simulink model "regulator_P_simulink"  (R2025b)
settings: Solver=VariableStepAuto  StartTime=0.0  StopTime=150  RelTol=1e-3
values from neighbouring files (symbols this model uses):
  Kp_Bode = mnoznik*ZapasWzmocnieniaBezwymiarowy_bode    (= 3.22827114517)    [Regulator_P.m]
  Kp_Tau_T = (0.3)/(Kr*(tau/T))    [Regulator_P.m]
  L1 = [3]    [Regulator_P.m]
  M1 = conv(m4,m5)    [Regulator_P.m]
settings Model: LastModifiedBy=mefir

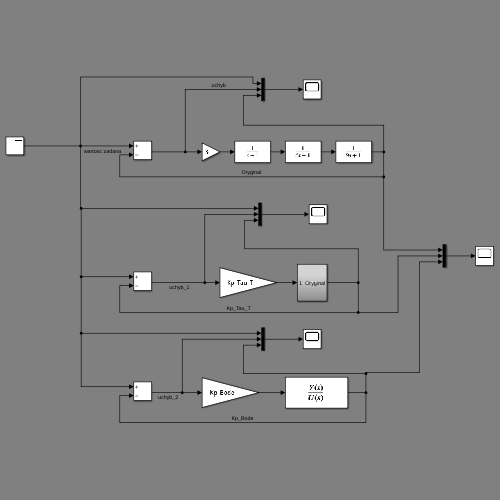
[thumbnail: Simulink's stored preview of the top-level diagram]
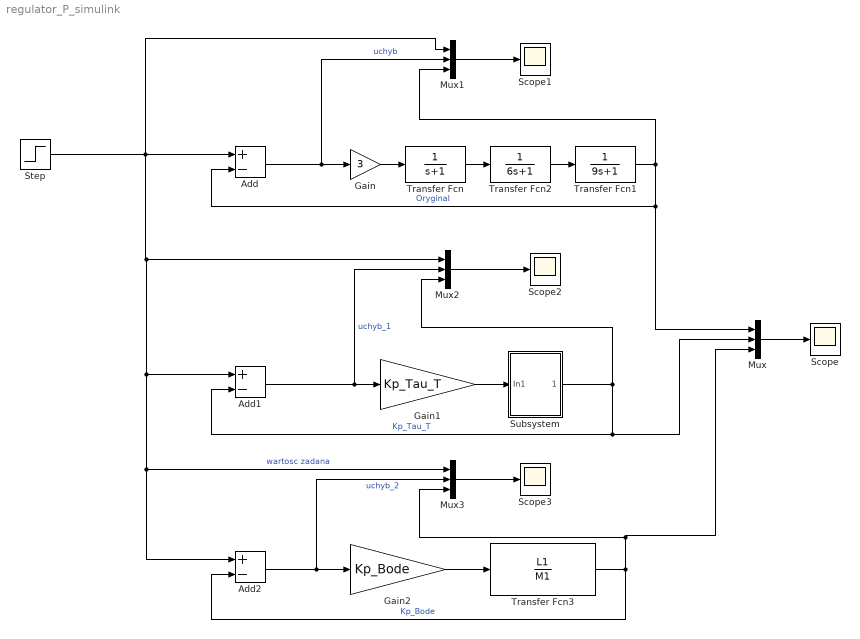
== system regulator_P_simulink ==
  Add : Sum  Inputs=+-
  Add1 : Sum  Inputs=+-
  Add2 : Sum  Inputs=+-
  Gain : Gain  Gain=3
  Gain1 : Gain  Gain=Kp_Tau_T
  Gain2 : Gain  Gain=Kp_Bode
  Mux{,1..3} (4 alike) : Mux  Inputs=3
  Scope{,1..3} (4 alike) : Scope
      Scope settings: ActiveDisplayYMinimum=-0.18004571836253325  ActiveDisplayYMaximum=1.6204114652627999
      Scope1 settings: ActiveDisplayYMinimum=-0.18004571836253325  ActiveDisplayYMaximum=1.6204114652627999
      Scope2 settings: ActiveDisplayYMinimum=-0.18004571836253325  ActiveDisplayYMaximum=1.6204114652627999  DataLoggingVariableName=ScopeData2
      Scope3 settings: ActiveDisplayYMinimum=-0.92077361092448817  ActiveDisplayYMaximum=2.8222475639378457  DataLoggingVariableName=ScopeData3
  Step : Step  Time=0  SampleTime=0
  Subsystem : Subsystem
  Transfer Fcn : TransferFcn  Denominator=[1 1]
  Transfer Fcn1 : TransferFcn  Denominator=[9 1]
  Transfer Fcn2 : TransferFcn  Denominator=[6 1]
  Transfer Fcn3 : TransferFcn  Numerator=L1  Denominator=M1
  wires:
  Transfer Fcn/1 -> Transfer Fcn2/1
  Transfer Fcn2/1 -> Transfer Fcn1/1
  Gain/1 -> Transfer Fcn/1
  Add/1 -> Mux1/2, Gain/1  "uchyb"
  Transfer Fcn1/1 -> Mux1/3, Mux/1, Add/2  "Oryginal"
  Add1/1 -> Mux2/2, Gain1/1  "uchyb_1"
  Gain1/1 -> Subsystem/1(In1)
  Subsystem/1(Oryginal) -> Mux2/3, Add1/2, Mux/2  "Kp_Tau_T"
  Step/1 -> Add/1, Mux2/1, Add1/1, Mux3/1, Add2/1, Mux1/1  "wartosc zadana"
  Add2/1 -> Mux3/2, Gain2/1  "uchyb_2"
  Transfer Fcn3/1 -> Add2/2, Mux3/3, Mux/3  "Kp_Bode"
  Mux/1 -> Scope/1
  Mux1/1 -> Scope1/1
  Gain2/1 -> Transfer Fcn3/1
  Mux2/1 -> Scope2/1
  Mux3/1 -> Scope3/1

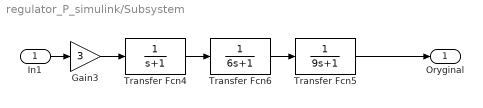
== system regulator_P_simulink/Subsystem ==
  In1 : Inport
  Gain3 : Gain  Gain=3
  Transfer Fcn4 : TransferFcn  Denominator=[1 1]
  Transfer Fcn5 : TransferFcn  Denominator=[9 1]
  Transfer Fcn6 : TransferFcn  Denominator=[6 1]
  Oryginal : Outport
  wires:
  Transfer Fcn4/1 -> Transfer Fcn6/1
  Transfer Fcn6/1 -> Transfer Fcn5/1
  Gain3/1 -> Transfer Fcn4/1
  Transfer Fcn5/1 -> Oryginal/1
  In1/1 -> Gain3/1
